simulink model "CHW2_Q9_Simulink"  (R2021b)
settings: Solver=VariableStepAuto  StartTime=0.0  StopTime=20.0  RelTol=1e-3
settings Model: Creator=Matin  LastModifiedBy=Matin

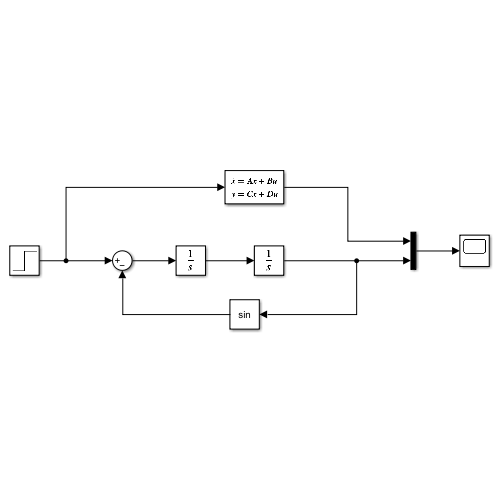
[thumbnail: Simulink's stored preview of the top-level diagram]
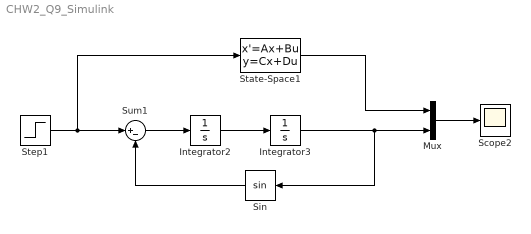
== system CHW2_Q9_Simulink ==
  Integrator2 : Integrator
  Integrator3 : Integrator
  Mux : Mux  Inputs=2
  Scope2 : Scope
  Sin : Trigonometry  OutputSignalType=real
  State-Space1 : StateSpace  A=[0 1;-1 0]  B=[0;1]  C=[1 0]  D=0  InitialCondition=0
  Step1 : Step  Time=0  After=0.1  SampleTime=0.0001
  Sum1 : Sum  Inputs=|+-
  wires:
  Sum1/1 -> Integrator2/1
  Step1/1 -> State-Space1/1, Sum1/1
  Integrator2/1 -> Integrator3/1
  Integrator3/1 -> Sin/1, Mux/2
  Sin/1 -> Sum1/2
  Mux/1 -> Scope2/1
  State-Space1/1 -> Mux/1
